simulink model "mitrule"  (R2022b)
settings: Solver=VariableStepAuto  StartTime=0.0  StopTime=300  FixedStep=0.1  RelTol=1e-3
values from neighbouring files (symbols this model uses):
  L_deltaa = ((rho*s*v^2*b)/2*I_xx)*c_ldeltaa    (= 0.0088445952)    [parameter.m]
  L_p = ((rho*s*v*b^2)/4*I_xx)*c_lp    (= -0.007578712512)    [parameter.m]
settings Model: Creator=110  LastModifiedBy=110

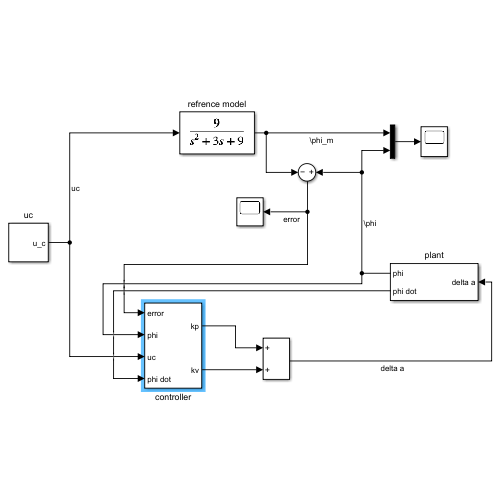
[thumbnail: Simulink's stored preview of the top-level diagram]
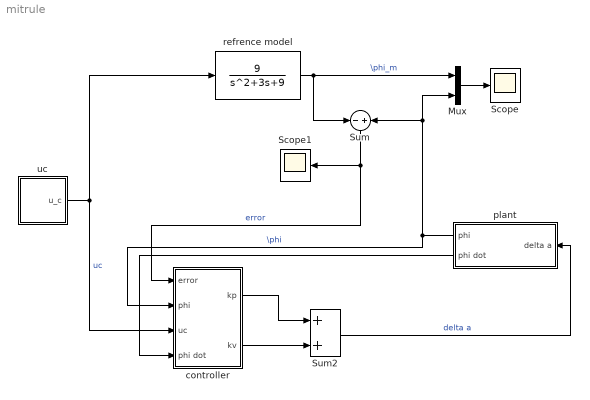
== system mitrule ==
  Mux : Mux  Inputs=2
  Scope : Scope
  Scope1 : Scope
  Sum : Sum  Inputs=-+
  Sum2 : Sum
  controller : Subsystem
  plant : Subsystem
  refrence model : TransferFcn  Numerator=9  Denominator=[1 3 9]
  uc : Subsystem
  wires:
  uc/1(u_c) -> controller/3(uc), refrence model/1  "uc"
  refrence model/1 -> Mux/1, Sum/1  "\\phi_m"
  Mux/1 -> Scope/1
  Sum/1 -> controller/1(error), Scope1/1  "error"
  controller/1(kp) -> Sum2/1
  controller/2(kv) -> Sum2/2
  Sum2/1 -> plant/1(delta a)  "delta a"
  plant/1(phi) -> Sum/2, Mux/2, controller/2(phi)  "\\phi"
  plant/2(phi dot) -> controller/4(phi dot)

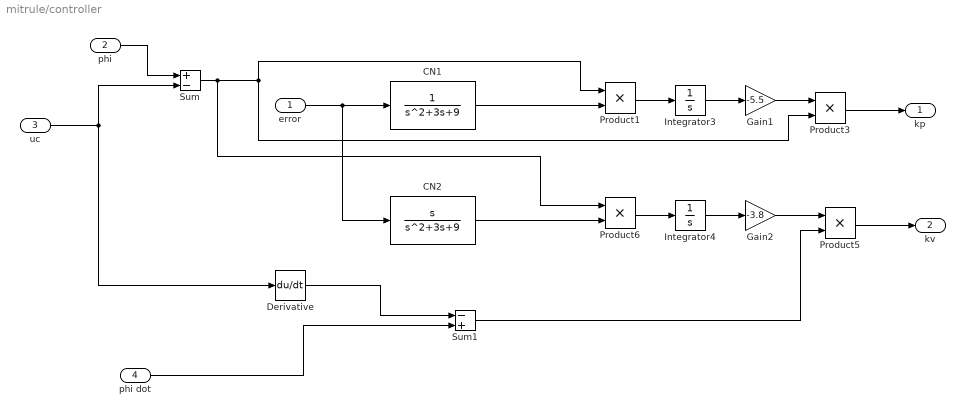
== system mitrule/controller ==
  error : Inport
  phi : Inport  Port=2
  uc : Inport  Port=3
  phi dot : Inport  Port=4
  CN1 : TransferFcn  Numerator=1  Denominator=[1 3 9]
  CN2 : TransferFcn  Numerator=[1 0]  Denominator=[1 3 9]
  Derivative : Derivative
  Gain1 : Gain  Gain=-5.5
  Gain2 : Gain  Gain=-3.8
  Integrator3 : Integrator
  Integrator4 : Integrator
  Product{1,3,5..6} (4 alike) : Product
  Sum : Sum  Inputs=+-
  Sum1 : Sum  Inputs=-+
  kp : Outport
  kv : Outport  Port=2
  wires:
  Gain2/1 -> Product5/1
  Integrator4/1 -> Gain2/1
  Integrator3/1 -> Gain1/1
  Gain1/1 -> Product3/1
  Product5/1 -> kv/1
  Product3/1 -> kp/1
  phi/1 -> Sum/1
  uc/1 -> Derivative/1, Sum/2
  Sum/1 -> Product6/1, Product3/2, Product1/1
  Product1/1 -> Integrator3/1
  Product6/1 -> Integrator4/1
  error/1 -> CN2/1, CN1/1
  CN2/1 -> Product6/2
  CN1/1 -> Product1/2
  phi dot/1 -> Sum1/2
  Derivative/1 -> Sum1/1
  Sum1/1 -> Product5/2

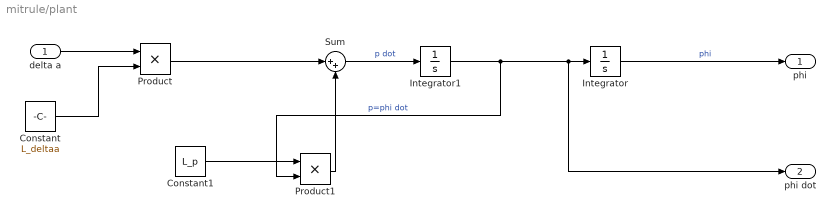
== system mitrule/plant ==
  delta a : Inport
  Constant : Constant  Value=L_deltaa
  Constant1 : Constant  Value=L_p
  Integrator : Integrator
  Integrator1 : Integrator
  Product : Product
  Product1 : Product
  Sum : Sum  Inputs=|++
  phi : Outport
  phi dot : Outport  Port=2
  wires:
  Integrator/1 -> phi/1  "phi"
  delta a/1 -> Product/1
  Constant/1 -> Product/2
  Product/1 -> Sum/1
  Product1/1 -> Sum/2
  Constant1/1 -> Product1/1
  Sum/1 -> Integrator1/1  "p dot"
  Integrator1/1 -> Product1/2, phi dot/1, Integrator/1  "p=phi dot"

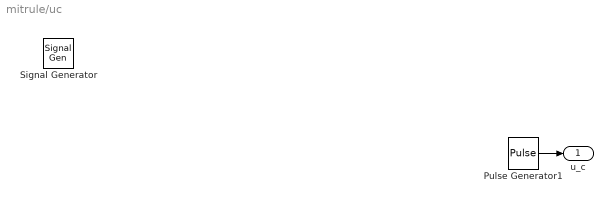
== system mitrule/uc ==
  Pulse Generator1 : DiscretePulseGenerator  PulseType=Time based  Amplitude=5  Period=20  PulseWidth=60
  Signal Generator : SignalGenerator  WaveForm=square  Amplitude=5  Units=rad/sec
  u_c : Outport
  wires:
  Pulse Generator1/1 -> u_c/1
